simulink model "testStateSpace"  (R2015a)
settings: Solver=ode4  StartTime=0.0  StopTime=50  FixedStep=0.01  RelTol=1e-3
values from neighbouring files (symbols this model uses):
  h0 = 20    [NastawyLQR.m]    (also in SzukanieNastaw.m; wskaznikJakosci.m)
  pompaPWM = ur(1)    [NastawyLQR.m]    (also in SzukanieNastaw.m; SzukanieStanuUstalonego.m = Nastawy(1); wskaznikJakosci.m = params(1))
  zaworPWM = ur(2)    [NastawyLQR.m]    (also in SzukanieNastaw.m; SzukanieStanuUstalonego.m = Nastawy(2); wskaznikJakosci.m = params(2))
undefined symbols (not defined in the file or in its folder): A, B, C, D
settings Model: Creator=konra  LastModifiedBy=konra

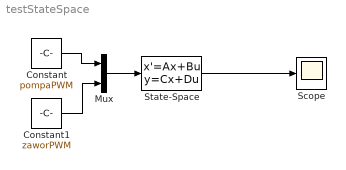
== system testStateSpace ==
  Constant : Constant  Value=pompaPWM
  Constant1 : Constant  Value=zaworPWM
  Mux : Mux  Inputs=2
  Scope : Scope
  State-Space : StateSpace  A=A  B=B  C=C  D=D  X0=h0
  wires:
  State-Space/1 -> Scope/1
  Constant1/1 -> Mux/2
  Mux/1 -> State-Space/1
  Constant/1 -> Mux/1
